simulink model "Prac_2_Q2_2"  (R2020a)
settings: Solver=VariableStepAuto  StartTime=0.0  StopTime=10.0  RelTol=1e-3
settings Model: Creator=kaibr  LastModifiedBy=kaibr

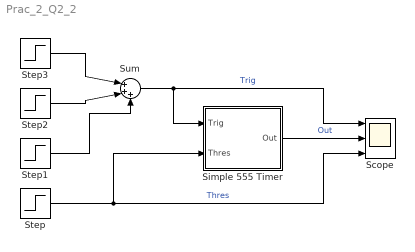
== system Prac_2_Q2_2 ==
  Scope : Scope  NumInputPorts=3
  Simple 555 Timer : Subsystem
  Step : Step  Time=3  After=10  SampleTime=0
  Step1 : Step  Time=4  After=10  SampleTime=0
  Step2 : Step  Time=2  After=-10  SampleTime=0
  Step3 : Step  After=10  SampleTime=0
  Sum : Sum  Inputs=|+++
  wires:
  Step/1 -> Scope/3, Simple 555 Timer/2(Thres)  "Thres"
  Simple 555 Timer/1(Out) -> Scope/2  "Out"
  Step3/1 -> Sum/1
  Step2/1 -> Sum/2
  Step1/1 -> Sum/3
  Sum/1 -> Scope/1, Simple 555 Timer/1(Trig)  "Trig"

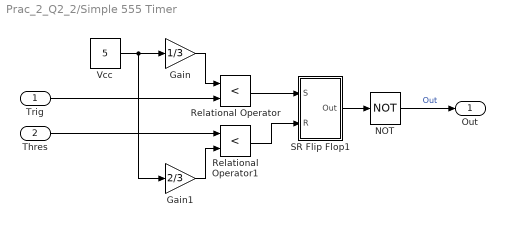
== system Prac_2_Q2_2/Simple 555 Timer ==
  Trig : Inport
  Thres : Inport  Port=2
  Gain : Gain  Gain=1/3
  Gain1 : Gain  Gain=2/3
  NOT : Logic  Operator=NOT  IconShape=distinctive  AllPortsSameDT=off  OutDataTypeStr=boolean
  Relational Operator : RelationalOperator  Operator=<  OutDataTypeStr=boolean  RndMeth=Simplest
  Relational Operator1 : RelationalOperator  Operator=<  OutDataTypeStr=boolean  RndMeth=Simplest
  SR Flip Flop1 : Subsystem
  Vcc : Constant  Value=5
  Out : Outport
  wires:
  Vcc/1 -> Gain1/1, Gain/1
  NOT/1 -> Out/1  "Out"
  Trig/1 -> Relational Operator/2
  Gain/1 -> Relational Operator/1
  SR Flip Flop1/1(Out) -> NOT/1
  Relational Operator/1 -> SR Flip Flop1/1(S)
  Thres/1 -> Relational Operator1/1
  Gain1/1 -> Relational Operator1/2
  Relational Operator1/1 -> SR Flip Flop1/2(R)

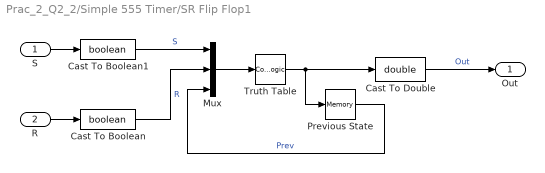
== system Prac_2_Q2_2/Simple 555 Timer/SR Flip Flop1 ==
  S : Inport
  R : Inport  Port=2
  Cast To Boolean : DataTypeConversion  OutDataTypeStr=boolean
  Cast To Boolean1 : DataTypeConversion  OutDataTypeStr=boolean
  Cast To Double : DataTypeConversion  OutDataTypeStr=double
  Mux : Mux  Inputs=3
  Previous State : Memory
  Truth Table : CombinatorialLogic  TruthTable=[0; 1; 0; 0; 1; 1; 0; 0]
  Out : Outport
  wires:
  Truth Table/1 -> Cast To Double/1, Previous State/1
  Previous State/1 -> Mux/3  "Prev"
  Mux/1 -> Truth Table/1
  Cast To Double/1 -> Out/1  "Out"
  S/1 -> Cast To Boolean1/1
  Cast To Boolean1/1 -> Mux/1  "S"
  R/1 -> Cast To Boolean/1
  Cast To Boolean/1 -> Mux/2  "R"
